simulink model "apsk16_pilot_phase_sync"  (Simulink 9.1)
settings: Solver=FixedStepDiscrete  StartTime=0.0  StopTime=inf  RelTol=1e-3
undefined symbols (not defined in the file): gcbh, i, rcfiltgaincompat
libraries: dspobslib x4, commfilt2 x2, commrandsrc2 x2, commchan3 x1, commrflib2 x1, commdigbbndpm3 x1, simulink x1
settings Model: SuppressorTable="22 serialization::archive 11 0 6 0 0 1 8 0 0 0 0 6 0 0 1 0 53 apsk16_pilot_phase_sync/QPSK Shedule/Counter Limited1 0 6 0 0 2 8 0 0 0 0 6 41 Simulink:DataType:WarningOverFlowDetected 0 0 0 6 0  0  0 0 0 0 8 20160608 0 0 0 15 23 17 0 1 40 SimulinkFixedPoint:util:Overflowoccurred 0 0 0  0  8 20160608 0 15 23 17 0 1"  Creator=Admin  LastModifiedBy=User
settings DataIOCC: LimitDataPoints=on  SignalLoggingSaveFormat=ModelDataLogs
settings OptimizationCC: ExpressionDepthLimit=2147483647  InitFltsAndDblsToZero=on
settings DebuggingCC: SolverPrmCheckMsg=warning  FcnCallInpInsideContextMsg=warning  StateNameClashWarn=warning

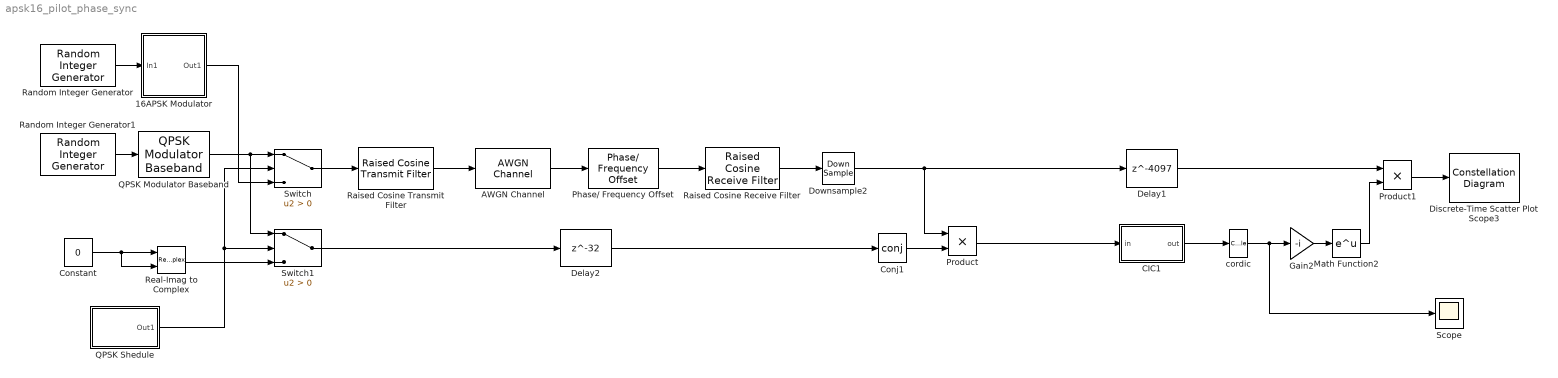
== system apsk16_pilot_phase_sync ==
  16APSK Modulator : Subsystem
  AWGN Channel : commchan3/AWGN Channel  InputProcessing=Columns as channels (frame based)  seed=67  noiseMode="Signal to noise ratio  (Eb/No)"  EbNodB=20  EsNodB=10  SNRdB=10  bitsPerSym=2  Ps=0.1250  Tsym=1  variance=1
  CIC1 : Subsystem
  Conj1 : Math  Operator=conj  SaturateOnIntegerOverflow=on
  Constant : Constant  Value=0
  Delay1 : Delay  DelayLength=4097  InitialCondition=0  InputProcessing=Inherited
  Delay2 : Delay  DelayLength=32  InitialCondition=0  InputProcessing=Inherited
  Discrete-Time Scatter Plot Scope3 : ConstellationDiagram  Tag=ScatterPlot
  Downsample2 : DownSample  N=8  InputProcessing=Inherited (this choice will be removed - see release notes)  RateOptions=Allow multirate processing
  Gain2 : Gain  Gain=-i  SaturateOnIntegerOverflow=on  OutDataTypeStr=Inherit: Same as input  ParamDataTypeStr=Inherit: Same as input
  Math Function2 : Math  SaturateOnIntegerOverflow=on
  Phase/ Frequency Offset : commrflib2/Phase// Frequency Offset  phaseOffset=0  freqPort=off  freqOffset=1e-5
      settings: SourceProductName=Communications System Toolbox
  Product : Product
  Product1 : Product
  QPSK Modulator Baseband : commdigbbndpm3/QPSK Modulator Baseband  InType=Integer  Enc=Gray  Ph=pi/4  outDtype=double  outWordLen=16  outUDDataType=sfix(16)  outFracLenMode=Best precision  outFracLen=15  outDataTypeStr=double  outLastDataTypeStr=double
  QPSK Shedule : Subsystem
  Raised Cosine Receive Filter : commfilt2/Raised Cosine Receive Filter  filtType=Square root  R=0.2  filtSpan=2*(16)  N=8  downFactor=1  downOffset=0  filterGain=rcfiltgaincompat(gcbh)  InputProcessing=Columns as channels (frame based)  RateOptions=Allow multirate processing  framing=Mute  checkCoeff=off  variableName=rcRxFilt  currentFiltSpan=2*(16)  D=16  inputOffset=0  sampMode=Mute  saveAsFlag=0  rateMode=Downsampling  checkGain=Normalized  launchFVT=off  roundingMode=Floor  overflowMode=off  coeffDataTypeStr=Inherit: Same word length as input  coeffMin=[]  coeffMax=[]  coeffLastDataTypeStr=Inherit: Same word length as input  accumDataTypeStr=Inherit: Same as product output  accumLastDataTypeStr=Inherit: Same as product output  outputDataTypeStr=Inherit: Same as accumulator  outputMin=[]  outputMax=[]  outputLastDataTypeStr=Inherit: Same as accumulator
  Raised Cosine Transmit Filter : commfilt2/Raised Cosine Transmit Filter  filtType=Square root  R=0.2  filtSpan=2*(16)  N=8  filterGain=rcfiltgaincompat(gcbh)  InputProcessing=Columns as channels (frame based)  RateOptions=Allow multirate processing  framing=Mute  checkCoeff=off  variableName=rcTxFilt  checkGain=Normalized  sampMode=Mute  saveAsFlag=0  currentFiltSpan=2*(16)  D=16  launchFVT=off  roundingMode=Floor  overflowMode=off  coeffDataTypeStr=Inherit: Same word length as input  coeffMin=[]  coeffMax=[]  coeffLastDataTypeStr=Inherit: Same word length as input  outputDataTypeStr=Inherit: Same as accumulator  outputMin=[]  outputMax=[]  outputLastDataTypeStr=Inherit: Same as accumulator
  Random Integer Generator : commrandsrc2/Random Integer Generator  mul=16  seed=37  Ts=1.  frameBased=off  sampPerFrame=1  orient=off  outDataType=double
  Random Integer Generator1 : commrandsrc2/Random Integer Generator  mul=4  seed=37  Ts=1.  frameBased=off  sampPerFrame=1  orient=off  outDataType=double
  Real-Imag to Complex : RealImagToComplex
  Scope : Scope
  Switch : Switch  Criteria=u2 > Threshold
  Switch1 : Switch  Criteria=u2 > Threshold
  cordic : ComplexToMagnitudeAngle  Output=Angle
  wires:
  Random Integer Generator/1 -> 16APSK Modulator/1(In1)
  Random Integer Generator1/1 -> QPSK Modulator Baseband/1
  Constant/1 -> Real-Imag to Complex/2, Real-Imag to Complex/1
  Math Function2/1 -> Product1/2
  Downsample2/1 -> Delay1/1, Product/1
  Delay1/1 -> Product1/1
  Switch/1 -> Raised Cosine Transmit Filter/1
  Raised Cosine Receive Filter/1 -> Downsample2/1
  Product/1 -> CIC1/1(in)
  cordic/1 -> Scope/1, Gain2/1
  Gain2/1 -> Math Function2/1
  CIC1/1(out) -> cordic/1
  Delay2/1 -> Conj1/1
  Phase/ Frequency Offset/1 -> Raised Cosine Receive Filter/1
  Raised Cosine Transmit Filter/1 -> AWGN Channel/1
  Conj1/1 -> Product/2
  AWGN Channel/1 -> Phase/ Frequency Offset/1
  Switch1/1 -> Delay2/1
  QPSK Shedule/1(Out1) -> Switch/2, Switch1/2
  QPSK Modulator Baseband/1 -> Switch1/1, Switch/1
  Real-Imag to Complex/1 -> Switch1/3
  16APSK Modulator/1(Out1) -> Switch/3
  Product1/1 -> Discrete-Time Scatter Plot Scope3/1

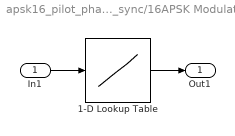
== system apsk16_pilot_phase_sync/16APSK Modulator ==
  In1 : Inport
  1-D Lookup Table : Lookup_n-D  NumberOfTableDimensions=1  BreakpointsForDimension1=[0:15]  Table=[0.8031+0.8031i 0.8031-0.8031i -0.8031+0.8031i -0.8031-0.8031i 1.0971+0.2940i 1.0971-0.2940i -1.0971+0.2940i -1.0971-0.2940i 0.2940+1.0971i 0.2940-1.0971i -0.2940+1.0971i -0.2940-1.0971i 0.2550+0.2550i 0.2550-0.2550i -0.2550+0.2550i -0.2550-0.2550i]  InterpMethod=Flat  ExtrapMethod=Clip  DiagnosticForOutOfRangeInput=Error  UseLastTableValue=on  InternalRulePriority=Speed  RndMeth=Simplest  InputSameDT=on
  Out1 : Outport
  wires:
  In1/1 -> 1-D Lookup Table/1
  1-D Lookup Table/1 -> Out1/1

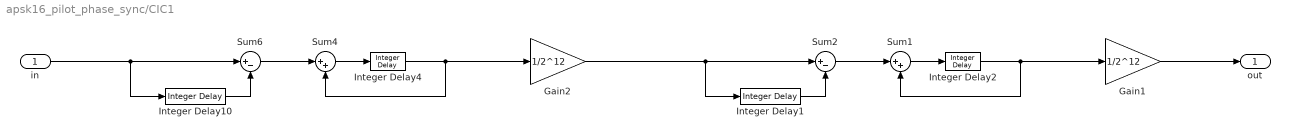
== system apsk16_pilot_phase_sync/CIC1 ==
  in : Inport
  Gain1 : Gain  Gain=1/2^12  SaturateOnIntegerOverflow=on  OutDataTypeStr=Inherit: Same as input  ParamDataTypeStr=Inherit: Same as input
  Gain2 : Gain  Gain=1/2^12  SaturateOnIntegerOverflow=on  OutDataTypeStr=Inherit: Same as input  ParamDataTypeStr=Inherit: Same as input
  Integer Delay1 : dspobslib/Integer Delay  delay=2^12  ic=0  reset_popup=None
      settings: SourceProductName=DSP System Toolbox  SourceProductBaseCode=DS
  Integer Delay10 : dspobslib/Integer Delay  delay=2^12  ic=0  reset_popup=None
      settings: SourceProductName=DSP System Toolbox  SourceProductBaseCode=DS
  Integer Delay2 : dspobslib/Integer Delay  delay=1  ic=0  reset_popup=None
      settings: SourceProductName=DSP System Toolbox  SourceProductBaseCode=DS
  Integer Delay4 : dspobslib/Integer Delay  delay=1  ic=0  reset_popup=None
      settings: SourceProductName=DSP System Toolbox  SourceProductBaseCode=DS
  Sum1 : Sum  Inputs=|++  SaturateOnIntegerOverflow=on  InputSameDT=on  OutDataTypeStr=Inherit: Same as first input
  Sum2 : Sum  Inputs=|+-  SaturateOnIntegerOverflow=on  InputSameDT=on  OutDataTypeStr=Inherit: Same as first input
  Sum4 : Sum  Inputs=|++  SaturateOnIntegerOverflow=on  InputSameDT=on  OutDataTypeStr=Inherit: Same as first input
  Sum6 : Sum  Inputs=|+-  SaturateOnIntegerOverflow=on  InputSameDT=on  OutDataTypeStr=Inherit: Same as first input
  out : Outport
  wires:
  in/1 -> Sum6/1, Integer Delay10/1
  Integer Delay10/1 -> Sum6/2
  Sum4/1 -> Integer Delay4/1
  Integer Delay4/1 -> Sum4/2, Gain2/1
  Sum6/1 -> Sum4/1
  Sum2/1 -> Sum1/1
  Gain2/1 -> Sum2/1, Integer Delay1/1
  Sum1/1 -> Integer Delay2/1
  Integer Delay2/1 -> Sum1/2, Gain1/1
  Integer Delay1/1 -> Sum2/2
  Gain1/1 -> out/1

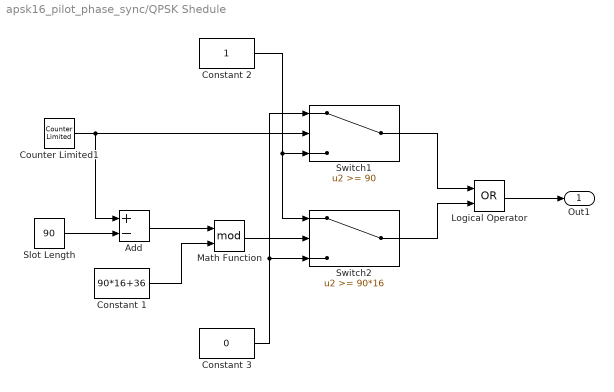
== system apsk16_pilot_phase_sync/QPSK Shedule ==
  Add : Sum  Inputs=+-
  Constant 1 : Constant  Value=90*16+36
  Constant 2 : Constant
  Constant 3 : Constant  Value=0
  Counter Limited1 : simulink/Sources/Counter Limited  uplimit=4140  tsamp=-1
  Logical Operator : Logic  Operator=OR  AllPortsSameDT=off  OutDataTypeStr=boolean
  Math Function : Math  Operator=mod  SaturateOnIntegerOverflow=on
  Slot Length : Constant  Value=90
  Switch1 : Switch  Threshold=90
  Switch2 : Switch  Threshold=90*16
  Out1 : Outport
  wires:
  Counter Limited1/1 -> Add/1, Switch1/2
  Slot Length/1 -> Add/2
  Add/1 -> Math Function/1
  Constant 1/1 -> Math Function/2
  Math Function/1 -> Switch2/2
  Constant 2/1 -> Switch1/3, Switch2/1
  Constant 3/1 -> Switch2/3, Switch1/1
  Switch1/1 -> Logical Operator/1
  Switch2/1 -> Logical Operator/2
  Logical Operator/1 -> Out1/1
